simulink model "psbcirc2ss_slk"  (Simulink 6.0)
settings: Solver=ode15s  SolverMode=SingleTasking  StartTime=0.0  StopTime=0.25  RelTol=1e-4  AbsTol=1e-6
values from neighbouring files (symbols this model uses):
  y = j*b    [etazline.m]
undefined symbols (not defined in the file or in its folder): A, B, C, D, x0
libraries: powerlib_models x2, powerlib_extras x1
settings Model: Creator=patrice  LastModifiedBy=batserve  ExtModeTrigMode=oneshot  ExtModeArmWhenConnect=off  ExtModeAutoUpdateStatusClock=off
settings DataIOCC: LimitDataPoints=off  SignalLoggingName=sigsOut
settings OptimizationCC: BlockReduction=off  BooleanDataType=off
settings DebuggingCC: SolverPrmCheckMsg=none
settings HardwareCC: TargetUnknown=on

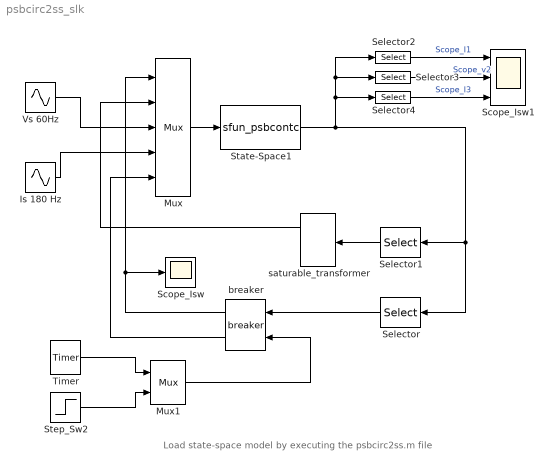
== system psbcirc2ss_slk ==
  note: Load state-space model by executing the psbcirc2ss.m file
  Is 180 Hz : Sin  Amplitude=2  Frequency=2*pi*180  Phase=-30*pi/180  SampleTime=0
  Mux : Mux  Inputs=[2 1 1 1 2]
  Mux1 : Mux  Inputs=2
  Scope_Isw : Scope
      settings: TickLabels=on  TimeRange=0.0001  YMin=-1  YMax=1  DataFormat=Array
  Scope_Isw1 : Scope  NumInputPorts=3
      settings: TickLabels=on  TimeRange=0.25  YMin=-20~-400~-400  YMax=10~200~200  DataFormat=Array
  Selector : Selector  Orientation=left  Elements=[1 2]  InputPortWidth=8
  Selector1 : Selector  Orientation=left  Elements=5  InputPortWidth=8
  Selector2 : Selector  Elements=6  InputPortWidth=8
  Selector3 : Selector  Elements=7  InputPortWidth=8
  Selector4 : Selector  Elements=8  InputPortWidth=8
  State-Space1 : S-Function  FunctionName=sfun_psbcontc  Parameters=A,B,C,D,x0,[0.1;0.1],y
  Step_Sw2 : Step  Time=0.05  SampleTime=0
  Timer : powerlib_extras/Control  Blocks/Timer  t=[0 100e-3 130e-3]  e=[1 0 1 ]
  Vs 60Hz : Sin  Amplitude=100  Frequency=2*pi*60  SampleTime=0
  breaker : powerlib_models/Continuous/breaker  Orientation=left  Nsw=2  istate=0  Rsw=1
  saturable_transformer : powerlib_models/Continuous/saturable_transformer  Orientation=left  isat=[-141.42135623731 -0.14142135623731 0.14142135623731 141.42135623731]  phisat=[-0.487671337918433 -0.450158158078553 0.450158158078553 0.487671337918433]  fluxinit=-0.270695162980763
  wires:
  Mux/1 -> State-Space1/1
  Step_Sw2/1 -> Mux1/2
  Mux1/1 -> breaker/2
  Timer/1 -> Mux1/1
  breaker/1 -> Scope_Isw/1, Mux/1
  saturable_transformer/1 -> Mux/2
  Vs 60Hz/1 -> Mux/3
  Is 180 Hz/1 -> Mux/4
  breaker/2 -> Mux/5
  Selector/1 -> breaker/1
  Selector1/1 -> saturable_transformer/1
  State-Space1/1 -> Selector/1, Selector1/1, Selector2/1, Selector3/1, Selector4/1
  Selector2/1 -> Scope_Isw1/1  "Scope_I1"
  Selector3/1 -> Scope_Isw1/2  "Scope_v2"
  Selector4/1 -> Scope_Isw1/3  "Scope_I3"
